simulink model "Experiment_1"  (R2018b)
settings: Solver=VariableStepAuto  StartTime=0.0  StopTime=1  RelTol=1e-3
libraries: commchan3 x1
settings Model: Creator=sangh  LastModifiedBy=sangh

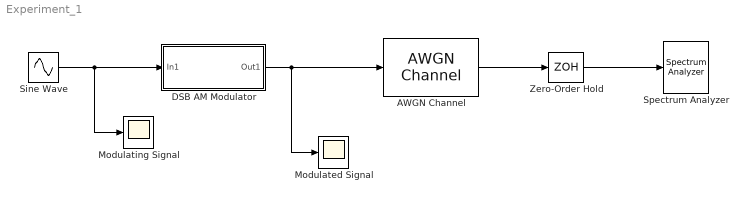
== system Experiment_1 ==
  AWGN Channel : commchan3/AWGN Channel  InputProcessing=Columns as channels (frame based)  seed=randseed  noiseMode=Variance from mask  EbNodB=10  EsNodB=10  SNRdB=10  bitsPerSym=1  Ps=1  Tsym=1  variance=0
  DSB AM Modulator : Subsystem
  Modulated Signal : Scope
  Modulating Signal : Scope
  Sine Wave : Sin  Frequency=2*pi*500  SampleTime=0.25e-6
  Spectrum Analyzer : SpectrumAnalyzer
  Zero-Order Hold : ZeroOrderHold  SampleTime=-1
  wires:
  Sine Wave/1 -> Modulating Signal/1, DSB AM Modulator/1(In1)
  DSB AM Modulator/1(Out1) -> AWGN Channel/1, Modulated Signal/1
  AWGN Channel/1 -> Zero-Order Hold/1
  Zero-Order Hold/1 -> Spectrum Analyzer/1

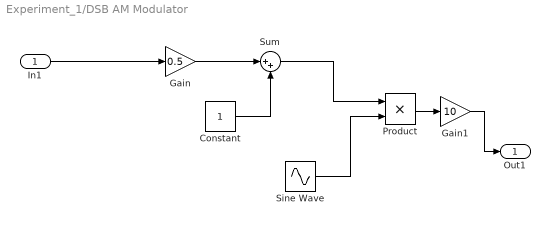
== system Experiment_1/DSB AM Modulator ==
  In1 : Inport
  Constant : Constant
  Gain : Gain  Gain=0.5
  Gain1 : Gain  Gain=10
  Product : Product
  Sine Wave : Sin  Frequency=2*pi*20e3  SampleTime=0.25e-6
  Sum : Sum  Inputs=|++
  Out1 : Outport
  wires:
  In1/1 -> Gain/1
  Gain/1 -> Sum/1
  Constant/1 -> Sum/2
  Sine Wave/1 -> Product/2
  Sum/1 -> Product/1
  Product/1 -> Gain1/1
  Gain1/1 -> Out1/1
